simulink model "simple_control_system_gain"  (R2021a)
settings: Solver=VariableStepAuto  StartTime=0.0  StopTime=10.0  RelTol=1e-3
settings Model: Creator=Beshary  LastModifiedBy=Beshary

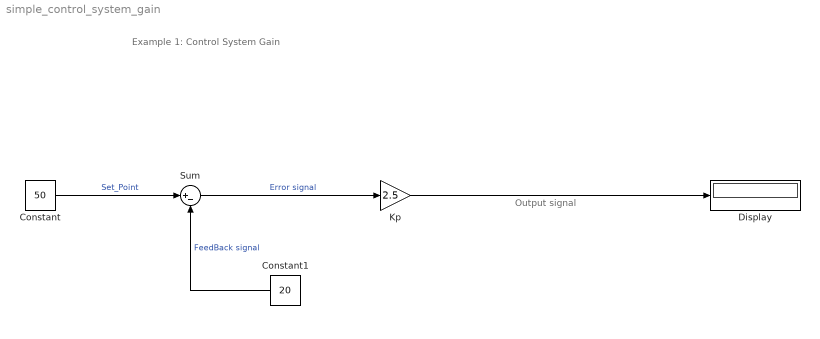
== system simple_control_system_gain ==
  note: Example 1: Control System Gain
  note: Output signal
  Constant : Constant  Value=50
  Constant1 : Constant  Value=20
  Display : Display
  Kp : Gain  Gain=2.5
  Sum : Sum  Inputs=|+-
  wires:
  Constant1/1 -> Sum/2  "FeedBack signal"
  Sum/1 -> Kp/1  "Error signal"
  Kp/1 -> Display/1
  Constant/1 -> Sum/1  "Set_Point"
